simulink model "SK_LPFsimulator_2018b"  (R2018b)
settings: Solver=FixedStepAuto  StartTime=0.0  StopTime=0.1  FixedStep=1e-6  MaxStep=3e-5  RelTol=1e-3  EnableMultiTasking=on
PreLoadFcn:
  | %% Global model parameters
  | fs = 1000; % A-to-D sampling rate
  | 
  | %% Filter design
  | f1 = 500; % Filter cut-off frequency
  | n = 4;    % Filter order
  | w1 = 2*pi*f1;
  | 
  | % [tmpB,tmpA] = besself(n,1); % Signal Processing Toolbox(TM)
  | tmpB = [0 0 0 0 1];
  | tmpA = [1.0000    3.1239    4.3916    3.2011    1.0000];
  | tmp_roots = roots(tmpA);
  | tcc1 = poly(tmp_roots(3:4));
  | a1 = tcc1(2);
  | b1 = tcc1(3);
  | tcc2 = poly(tmp_roots(1:2));
  | a2 = tcc2(2);
  | b2 = tcc2(3);
  | 
  | %% Filter implementation
  | R = 1e4;  % Resistance value
  | % Stage 1
  | C1 = a1/(2*b1);
  | C2 = 1/(b1*C1);
  | C1_1 = C1/( R*w1 );
  | C2_1 = C2/( R*w1 );
  | % Stage 2
  | C1 = a2/(2*b2);
  | C2 = 1/(b2*C1);
  | C1_2 = C1/( R*w1 );
  | C2_2 = C2/( R*w1 );
libraries: fl_lib x8, elec_lib x4, nesl_utility x3
CloseFcn:
  | try,close(h1_elec_a2d_sd_anti_alias),end
  | clear h1_elec_a2d_sd_anti_alias
  | 
  | 
  | clear simlog_elec_a2d_sd_anti_alias
  | clear logsout_elec_a2d_sd_anti_alias
  | clear C1 C1_1 C1_2 C2 C2_1 C2_2 R a1 a2 b1 b2 f1 fs n tcc1 tcc2 tmpA tmpB tmp_roots vOut w1
Description:
  | Analog Anti-Aliasing Filter
  | 
  | Copyright 2008-2018 The MathWorks, Inc.
settings Model: Creator=MathWorks  LastModifiedBy=yusuke
settings DataIOCC: MaxDataPoints=75000  SaveFormat=Array  SignalLoggingSaveFormat=ModelDataLogs  SaveOutput=off  SignalLogging=off  DSMLogging=off  SaveTime=off  SignalLoggingName=logsout_elec_a2d_sd_anti_alias
settings OptimizationCC: ExpressionDepthLimit=2147483647  LifeSpan=inf
settings DebuggingCC: UnderspecifiedInitializationDetection=Classic  MergeDetectMultiDrivingBlocksExec=none  SolverPrmCheckMsg=warning  FcnCallInpInsideContextMsg=warning  StateNameClashWarn=warning  SFUnexpectedBacktrackingDiag=warning  SFNoUnconditionalDefaultTransitionDiag=warning  SFExecutionAtInitializationDiag=none
settings HardwareCC: ProdBitPerPointer=32  ProdBitPerSizeT=32  ProdBitPerPtrDiffT=32  ProdLargestAtomicFloat=None  ProdIntDivRoundTo=Undefined  ProdEndianess=Unspecified  ProdWordSize=32  ProdHWDeviceType=32-bit Generic
settings ModelReferenceCC: PropagateSignalLabelsOutOfModel=off
settings SFSimCC: SimUseLocalCustomCode=off
settings RTWCC: RTWUseLocalCustomCode=off
settings CodeAppCC: StateflowObjectComments=on
settings GRTTargetCC: TargetLangStandard=C89/C90 (ANSI)  CombineOutputUpdateFcns=off  GRTInterface=on
settings ConfigComp: CovMetricSettings=dw  CovHtmlReporting=on  CovSaveCumulativeToWorkspaceVar=on  CovSaveSingleToWorkspaceVar=on  CovExternalEMLEnable=off  CovSFcnEnable=off
settings SimscapeCC: SimscapeLogType=all  SimscapeLogSimulationStatistics=on  SimscapeLogName=simlog_elec_a2d_sd_anti_alias  SimscapeLogDataHistory=75000

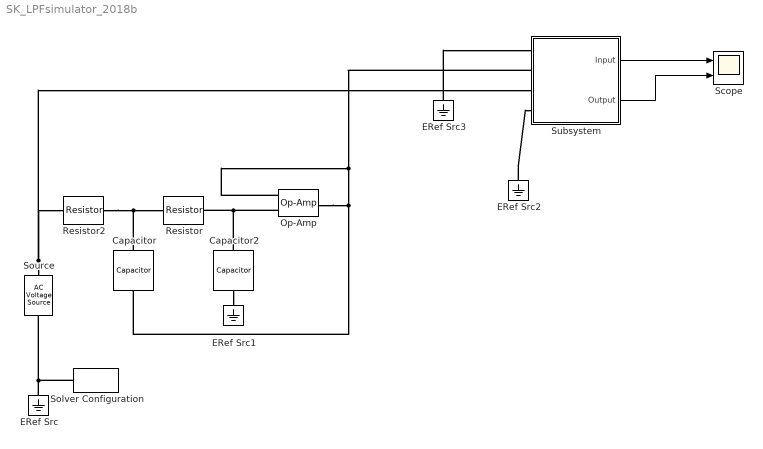
== system SK_LPFsimulator_2018b ==
  Capacitor : elec_lib/Passive Devices/Capacitor  enable_table=0  c=10 nF  Cvec=[1e-05, 1e-06] F  Vvec=[0, 10] V  CV_table_symmetry=1  C_tol=5  enable_C_tol=0  tol_distribution=1  nSigma=4  r=1e-6 Ohm  g=0 1/Ohm  enable_operating_limits=0  operating_limit_action=2  max_working_voltage_range=[-25, 25] V  power_rating=1 W  enable_faults=0  fault_action=1  Cscale_faulted=100  R_faulted=1e-3 Ohm  G_faulted=0 1/Ohm  tau_fault=1e-3 s  enable_temporal_fault=0  t_fault=1 s  enable_behavioral_fault=0  max_permissible_voltage_range=[-100, 100] V  t_fail_on_voltage=1 s  i_specify=off  i_priority=None  i=0 A  i_nominal_specify=off  i_nominal_unit=A  i_nominal_value=1  v_specify=off  v_priority=None  v=0 V  v_nominal_specify=off  v_nominal_unit=V  v_nominal_value=1  vc_specify=off  vc_priority=High  vc=0 V  vc_nominal_specify=off  vc_nominal_unit=V  vc_nominal_value=1
  Capacitor2 : elec_lib/Passive Devices/Capacitor  enable_table=0  c=10 nF  Cvec=[1e-05, 1e-06] F  Vvec=[0, 10] V  CV_table_symmetry=1  C_tol=5  enable_C_tol=0  tol_distribution=1  nSigma=4  r=1e-6 Ohm  g=0 1/Ohm  enable_operating_limits=0  operating_limit_action=2  max_working_voltage_range=[-25, 25] V  power_rating=1 W  enable_faults=0  fault_action=1  Cscale_faulted=100  R_faulted=1e-3 Ohm  G_faulted=0 1/Ohm  tau_fault=1e-3 s  enable_temporal_fault=0  t_fault=1 s  enable_behavioral_fault=0  max_permissible_voltage_range=[-100, 100] V  t_fail_on_voltage=1 s  i_specify=off  i_priority=None  i=0 A  i_nominal_specify=off  i_nominal_unit=A  i_nominal_value=1  v_specify=off  v_priority=None  v=0 V  v_nominal_specify=off  v_nominal_unit=V  v_nominal_value=1  vc_specify=off  vc_priority=High  vc=0 V  vc_nominal_specify=off  vc_nominal_unit=V  vc_nominal_value=1
  ERef Src{,1..3} (4 alike) : fl_lib/Electrical/Electrical Elements/Electrical Reference
      settings: SourceProductName=Foundation Library
  Op-Amp : fl_lib/Electrical/Electrical Elements/Op-Amp  outI_specify=off  outI_priority=None  outI=0 A  outI_nominal_specify=off  outI_nominal_unit=A  outI_nominal_value=1
  Resistor : elec_lib/Passive Devices/Resistor  R=10 kOhm  R_tol=5  enable_R_tol=0  tol_distribution=1  nSigma=4  enable_operating_limits=0  operating_limit_action=2  max_working_voltage=100 V  power_rating=1 W  enable_faults=0  fault_action=1  R_faulted=inf Ohm  enable_temporal_fault=0  t_fault=1 s  enable_behavioral_fault=0  max_permissible_current=1 A  t_fail_on_current=1 s  noise_mode=0  sample_time=1e-3 s  repeatability=1  auto_seed=3521792535  user_seed=0  Tdevice=25 degC  alpha=3.93e-3 1/K  Tmeas=25 degC  thermal_mass=100 J/K  power_derating_T1=70 degC  power_derating_T2=155 degC  operating_temperature_range_vec=[-50, 150] degC  temperature_specify=off  temperature_priority=High  temperature=298.15 K  temperature_nominal_specify=off  temperature_nominal_unit=K  temperature_nominal_value=1
  Resistor2 : elec_lib/Passive Devices/Resistor  R=10 kOhm  R_tol=5  enable_R_tol=0  tol_distribution=1  nSigma=4  enable_operating_limits=0  operating_limit_action=2  max_working_voltage=100 V  power_rating=1 W  enable_faults=0  fault_action=1  R_faulted=inf Ohm  enable_temporal_fault=0  t_fault=1 s  enable_behavioral_fault=0  max_permissible_current=1 A  t_fail_on_current=1 s  noise_mode=0  sample_time=1e-3 s  repeatability=1  auto_seed=1750711121  user_seed=0  Tdevice=25 degC  alpha=3.93e-3 1/K  Tmeas=25 degC  thermal_mass=100 J/K  power_derating_T1=70 degC  power_derating_T2=155 degC  operating_temperature_range_vec=[-50, 150] degC  temperature_specify=off  temperature_priority=High  temperature=298.15 K  temperature_nominal_specify=off  temperature_nominal_unit=K  temperature_nominal_value=1
  Scope : Scope  NumInputPorts=2
  Solver Configuration : nesl_utility/Solver Configuration  PhysicalDomain=network_engine_domain  SubClassName=solver  LeftPortType=input  RightPortType=generic  Tones=[]  Harmonics=[]  SimulateNoise=off  Profile=off  UseLocalSampling=off  EnableSwitchedLinearOptims=on  FrequencyDomain=off  UseCCode=off  RelTol=0.001  AbsTol=1e-06  MinStep=1e-09  ToWorkspace=off  RevertToSquareIcSolve=off  NumHomotopyIterations=100  PhasorMode=off  PhasorModeNumHarmonics=1  DoDC=off  ResidualTolerance=1e-9  UseLocalSolver=off  LocalSolverChoice=NE_BACKWARD_EULER_ADVANCER  LocalSolverSampleTime=1e-6  DoFixedCost=off  MaxNonlinIter=3  MaxModeIter=2  LinearAlgebra=auto  EquationFormulation=NE_TIME_EF  DelaysMemoryBudget=1024  AutomaticFiltering=on  FilteringTimeConstant=0.001  PartitionStorageMethod=AS_NEEDED  PartitionMemoryBudget=1024
  Source : fl_lib/Electrical/Electrical Sources/AC Voltage Source  amp=10 V  shift=0 deg  frequency=freqParam Hz  omega=0 rad/s
      settings: SourceProductName=Foundation Library
      settings: AttributesFormatString=|
      | %<amp> %<amp_unit>
      | %<frequency> %<frequency_unit>
  Subsystem : Subsystem
  wires:
  Subsystem/1(Input) -> Scope/1
  Subsystem/2(Output) -> Scope/2
  connections:
  Source/LConn1 -- Resistor2/LConn1 -- Subsystem/LConn3
  ERef Src/LConn1 -- Solver Configuration/RConn1 -- Source/RConn1
  Subsystem/LConn2 -- Op-Amp/RConn1 -- Capacitor/RConn1 -- Op-Amp/LConn2
  Capacitor2/RConn1 -- ERef Src1/LConn1
  Resistor2/RConn1 -- Capacitor/LConn1 -- Resistor/LConn1
  ERef Src3/LConn1 -- Subsystem/LConn1
  ERef Src2/LConn1 -- Subsystem/LConn4
  Capacitor2/LConn1 -- Op-Amp/LConn1 -- Resistor/RConn1

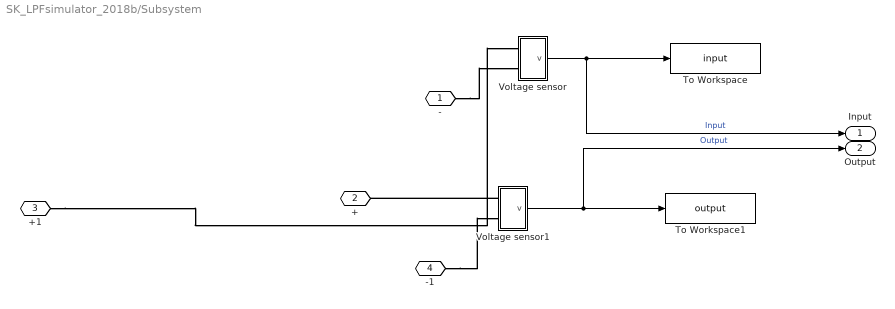
== system SK_LPFsimulator_2018b/Subsystem ==
  To Workspace : ToWorkspace  VariableName=input  SaveFormat=Timeseries  SampleTime=-1
  To Workspace1 : ToWorkspace  VariableName=output  SaveFormat=Timeseries  SampleTime=-1
  Voltage sensor : Subsystem
      settings: CopyFcn=set_param(gcb,'LinkStatus','none')
  Voltage sensor1 : Subsystem
      settings: CopyFcn=set_param(gcb,'LinkStatus','none')
  - : PMIOPort  Side=Left
  + : PMIOPort  Port=2  Side=Left
  +1 : PMIOPort  Port=3  Side=Left
  -1 : PMIOPort  Port=4  Side=Left
  Input : Outport  VectorParamsAs1DForOutWhenUnconnected=on
  Output : Outport  Port=2  VectorParamsAs1DForOutWhenUnconnected=on
  wires:
  Voltage sensor1/1(v) -> Output/1, To Workspace1/1  "Output"
  Voltage sensor/1(v) -> Input/1, To Workspace/1  "Input"
  connections:
  -1/RConn1 -- Voltage sensor1/LConn2
  -/RConn1 -- Voltage sensor/LConn2
  Voltage sensor1/LConn1 -- +/RConn1
  +1/RConn1 -- Voltage sensor/LConn1

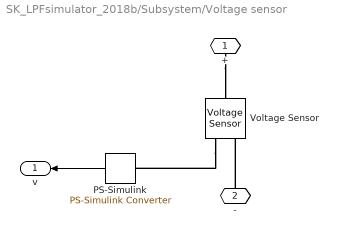
== system SK_LPFsimulator_2018b/Subsystem/Voltage sensor ==
  PS-Simulink : nesl_utility/PS-Simulink Converter  PhysicalDomain=network_engine_domain  SubClassName=ps_output  LeftPortType=input  RightPortType=output  PseudoPeriodic=off  Frequencies=[]  Unit=V  AffineConversion=off
  Voltage Sensor : fl_lib/Electrical/Electrical Sensors/Voltage Sensor
      settings: SourceProductName=Foundation Library
  + : PMIOPort  Side=Left
  - : PMIOPort  Port=2  Side=Left
  v : Outport
  wires:
  PS-Simulink/1 -> v/1
  connections:
  -/RConn1 -- Voltage Sensor/RConn2
  +/RConn1 -- Voltage Sensor/LConn1
  Voltage Sensor/RConn1 -- PS-Simulink/LConn1

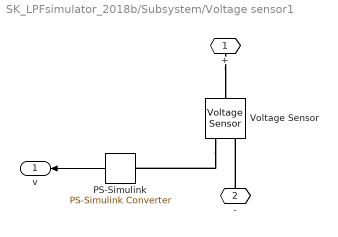
== system SK_LPFsimulator_2018b/Subsystem/Voltage sensor1 ==
  PS-Simulink : nesl_utility/PS-Simulink Converter  PhysicalDomain=network_engine_domain  SubClassName=ps_output  LeftPortType=input  RightPortType=output  PseudoPeriodic=off  Frequencies=[]  Unit=V  AffineConversion=off
  Voltage Sensor : fl_lib/Electrical/Electrical Sensors/Voltage Sensor
      settings: SourceProductName=Foundation Library
  + : PMIOPort  Side=Left
  - : PMIOPort  Port=2  Side=Left
  v : Outport
  wires:
  PS-Simulink/1 -> v/1
  connections:
  -/RConn1 -- Voltage Sensor/RConn2
  +/RConn1 -- Voltage Sensor/LConn1
  Voltage Sensor/RConn1 -- PS-Simulink/LConn1
